simulink model "finalMinhtest3105Part2"  (R2022b)
settings: Solver=VariableStepAuto  StartTime=0.0  StopTime=60  FixedStep=0.001  RelTol=1e-3
undefined symbols (not defined in the file): h, km, m, s, smiData, X, Y, Z
libraries: sm_lib x332, nesl_utility x27, aerolibconvert2 x13, simulink_extras x12, autolibshared x3, simulink x2
(part 1 of 8)
settings Model: Creator=dangm  LastModifiedBy=Lenovo
settings SolverCC: ZeroCrossAlgorithm=Adaptive  AlgebraicLoopSolver=LineSearch
settings DebuggingCC: IgnoredZcDiagnostic=none  UnconnectedInputMsg=warning  UnconnectedOutputMsg=warning  UnconnectedLineMsg=warning  SFMachineParentedDataDiag=warning
settings ModelReferenceCC: EnableRefExpFcnMdlSchedulingChecks=on

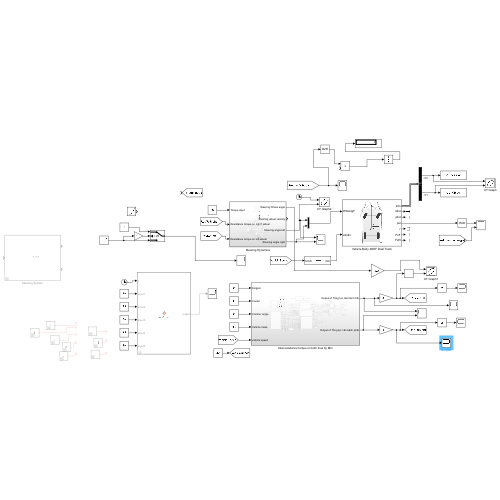
[thumbnail: Simulink's stored preview of the top-level diagram]
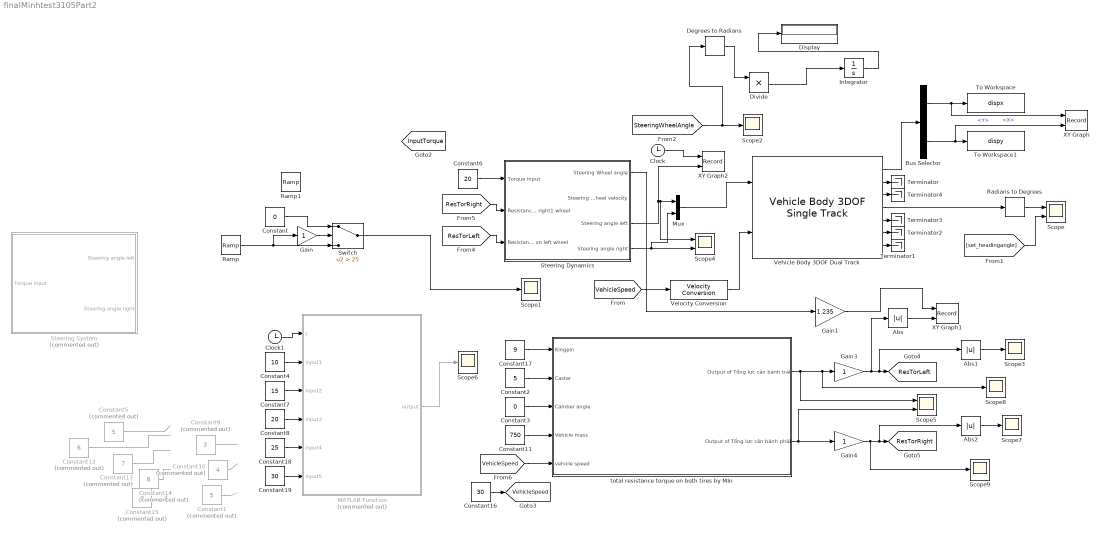
== system finalMinhtest3105Part2 ==
  Abs : Abs  SaturateOnIntegerOverflow=off
  Abs1 : Abs  SaturateOnIntegerOverflow=off
  Abs2 : Abs  SaturateOnIntegerOverflow=off
  Bus Selector : BusSelector  OutputSignals=InertFrm.Cg.Disp.X,InertFrm.Cg.Disp.Y
  Clock : Clock
  Clock1 : Clock
  Constant : Constant  Value=0
  Constant1 : Constant  Commented=on  Value=5
  Constant10 : Constant  Commented=on  Value=4
  Constant11 : Constant  Value=750
  Constant12 : Constant  Commented=on  Value=6
  Constant13 : Constant  Commented=on  Value=7
  Constant14 : Constant  Commented=on  Value=8
  Constant15 : Constant  Commented=on  Value=9
  Constant16 : Constant  Value=30
  Constant17 : Constant  Value=9
  Constant18 : Constant  Value=25
  Constant19 : Constant  Value=30
  Constant2 : Constant  Value=5
  Constant3 : Constant  Value=0
  Constant4 : Constant  Value=10
  Constant5 : Constant  Commented=on  Value=5
  Constant6 : Constant  Value=20
  Constant7 : Constant  Value=15
  Constant8 : Constant  Value=20
  Constant9 : Constant  Commented=on  Value=3
  Degrees to Radians : simulink_extras/Transformations/Degrees to Radians
  Display : Display
  Divide : Product  Inputs=**
  Gain : Gain
  Gain1 : Gain  Gain=1.235
  Gain3 : Gain
  Gain4 : Gain
  Integrator : Integrator
  MATLAB Function : MATLAB Function  Commented=on  TreatAsAtomicUnit=on
  Mux : Mux  Inputs=2
  Radians to Degrees : simulink_extras/Transformations/Radians to Degrees
  Ramp : simulink/Sources/Ramp  slope=1  start=0  InitialOutput=0
  Ramp1 : simulink/Sources/Ramp  slope=0.01  start=0  InitialOutput=0
  Scope : Scope  NumInputPorts=2
  Scope{1..3,6..9} (7 alike) : Scope
  Scope4 : Scope  NumInputPorts=2
  Scope5 : Scope  NumInputPorts=2
  Steering Dynamics : Subsystem
  Steering System : Subsystem  Commented=on
      mask Display: image('D:\MATLAB Projects\MATLAB_EPS_Complete_09_05\CapsoneProject\duy\mask\power-steering-2255498-1882000.png'); % Use "Edit Image" on toolstrip to change.
  Switch : Switch  Criteria=u2 > Threshold  Threshold=25  SaturateOnIntegerOverflow=off  InputSameDT=off
  Terminator{,1..4} (5 alike) : Terminator
  To Workspace : ToWorkspace  VariableName=dispx  SaveFormat=Structure With Time  SampleTime=-1
  To Workspace1 : ToWorkspace  VariableName=dispy  SaveFormat=Structure With Time  SampleTime=-1
  Vehicle Body 3DOF Dual Track : autolibshared/Vehicle Body 3DOF Single Track  trackMode=Dual  inputMode=External longitudinal velocity  frontSteerMode=on  rearSteerMode=off  windMode=off  muMode=off  extFMode=off  extMMode=off  htchFMode=off  htchMMode=off  extXo=off  extpsio=off  extxdoto=off  extro=off  extYo=off  extTamb=off  extydoto=off  aMode=2  NF=2  NR=2  m=1520  a=1.4  b=1.4  h=0.35  dh=1  hh=0.2  X_o=0  xdot_o=0  CalphaMode=off  sigmaMode=on  d=0  hl=0  w=[1.4,1.4]  Cy_f=12e3  Cy_r=11e3  sigma_f=.1  sigma_r=.1  alpha_f_brk=[-.1 .1]  Cy_f_data=[-9e3 9e3]  alpha_r_brk=[-.1 .1]  Cy_r_data=[-9e3 9e3]  Y_o=0  ydot_o=0  Izz=4000  psi_o=0  r_o=0  Af=2  Cd=.3  Cl=.1  Cpm=.1  beta_w=[0:0.01:0.3]  Cs=[0:0.03:0.9]  Cym=[0:0.01:0.3]  Pabs=101325  Tair=273  g=9.81  mu=1  xdot_tol=.01  Fznom=5000  Fxtire_sat=7e4  Fytire_sat=7e4  longOff=0  latOff=0  vertOff=0  wrapAng=off
  Velocity Conversion : aerolibconvert2/Velocity Conversion  IU=km/h  OU=m/s
  XY Graph : Record  FileSettingsInternal="{\"entries\":[{\"content\":{\"excelSettings\":{\"content\":{},\"type\":\"Streamout.ExcelSettings\"}},\"type\":\"Streamout.FileSettingStorage\",\"uuid\":\"8bd62942-ac25-41b1-a812-78b271daa7eb\"}],\"packageUris\":[\"http://schema.mathworks.com/mf0/streamout_blocks/R2020a\"],\"version\":\"1.0\"}"  Layout=[1 1]  SignalsInternal="{\"entries\":[{\"content\":{\"signals\":[{\"content\":{\"blockPath\":[\"FinalTest16_05Long32019b/XY Graph\"],\"channel\":[],\"dimensions\":[1],\"domain\":\"FinalTest16_05Long32019b/XY Graph\",\"lineColor\":\"#a2142f\",\"plots\":[1],\"port\":1,\"sid\":[\"\"],\"signalID\":18325,\"signalName\":\"<X>\"},\"type\":\"RecordBlkView.Signal\",\"uuid\":\"2b0177d6-e985-4d5a-bed9-d4c24acd87c5\"},{\"content\":{\"blockPath\":[\"FinalTest16_05Long32019b/XY Graph\"],\"channel\":[],\"dimensions\":[1],\"domain\":\"FinalTest16_05Long32019b/XY Graph\",\"lineColor\":\"#139fff\",\"plots\":[1],\"port\":2,\"sid\":[\"\"],\"signalID\":18329,\"signalName\":\"<Y>\"},\"type\":\"RecordBlkView.Signal\",\"uuid\":\"3202ecd1-4493-4db3-ae2f-ac69954db6bf\"}]},\"type\":\"RecordBlkView.InputSignals\",\"uuid\":\"6c82ded1-8226-4c26-a1f0-daf373c2f201\"}],\"packageUris\":[\"http://schema.mathworks.com/mf0/streamout_blocks/R2020a\"],\"version\":\"1.0\"}"  VisualizationBindings="{\"xyplotplugin\":{\"info\":[{\"series\":[{\"bindingParametersList\":[{\"parameter\":\"X-Axis\",\"signalID\":18325,\"signalName\":\"<X>\"},{\"parameter\":\"Y-Axis\",\"signalID\":18329,\"signalName\":\"<Y>\"}],\"seriesID\":52564}],\"subplotID\":1}]}}"  CompatibilityTag=XY  st=-1
  XY Graph1 : Record  FileSettingsInternal="{\"entries\":[{\"content\":{\"excelSettings\":{\"content\":{},\"type\":\"Streamout.ExcelSettings\"}},\"type\":\"Streamout.FileSettingStorage\",\"uuid\":\"d249e66b-4ac3-43e9-8db5-f8051359078a\"}],\"packageUris\":[\"http://schema.mathworks.com/mf0/streamout_blocks/R2020a\"],\"version\":\"1.0\"}"  Layout=[1 1]  SignalsInternal="{\"entries\":[{\"content\":{\"signals\":[{\"content\":{\"blockPath\":[\"FinalTest16_05Long32019b/XY Graph1\"],\"channel\":[],\"dimensions\":[1],\"domain\":\"FinalTest16_05Long32019b/XY Graph1\",\"lineColor\":\"#a2142f\",\"plots\":[1],\"port\":1,\"sid\":[\"\"],\"signalID\":18333,\"signalName\":\"Gain1\"},\"type\":\"RecordBlkView.Signal\",\"uuid\":\"ae25a6cb-4a64-4b64-b147-bb834be32e30\"},{\"content\":{\"blockPath\":[\"FinalTest16_05Long32019b/XY Graph1\"],\"channel\":[],\"dimensions\":[1],\"domain\":\"FinalTest16_05Long32019b/XY Graph1\",\"lineColor\":\"#139fff\",\"plots\":[1],\"port\":2,\"sid\":[\"\"],\"signalID\":18337,\"signalName\":\"Abs\"},\"type\":\"RecordBlkView.Signal\",\"uuid\":\"6c87c872-6dc0-4e7a-a83c-45ce04c5dd01\"}]},\"type\":\"RecordBlkView.InputSignals\",\"uuid\":\"a428bf55-466d-414c-9a8e-740befd34512\"}],\"packageUris\":[\"http://schema.mathworks.com/mf0/streamout_blocks/R2020a\"],\"version\":\"1.0\"}"  VisualizationBindings="{\"xyplotplugin\":{\"info\":[{\"series\":[{\"bindingParametersList\":[{\"parameter\":\"X-Axis\",\"signalID\":18333,\"signalName\":\"Gain1\"},{\"parameter\":\"Y-Axis\",\"signalID\":18337,\"signalName\":\"Abs\"}],\"seriesID\":19294}],\"subplotID\":1}]}}"  CompatibilityTag=XY  st=-1
  XY Graph2 : Record  FileSettingsInternal="{\"entries\":[{\"content\":{\"excelSettings\":{\"content\":{},\"type\":\"Streamout.ExcelSettings\"}},\"type\":\"Streamout.FileSettingStorage\",\"uuid\":\"ccaa301e-d718-420b-80cc-2ff8462626e4\"}],\"packageUris\":[\"http://schema.mathworks.com/mf0/streamout_blocks/R2020a\"],\"version\":\"1.0\"}"  Layout=[1 1]  SignalsInternal="{\"entries\":[{\"content\":{\"signals\":[{\"content\":{\"blockPath\":[\"FinalTest16_05Long32019b/XY Graph2\"],\"channel\":[],\"dimensions\":[1],\"domain\":\"FinalTest16_05Long32019b/XY Graph2\",\"lineColor\":\"#a2142f\",\"plots\":[1],\"port\":1,\"sid\":[\"\"],\"signalID\":18341,\"signalName\":\"Clock\"},\"type\":\"RecordBlkView.Signal\",\"uuid\":\"91adbf16-523e-4284-a861-e31794318eab\"},{\"content\":{\"blockPath\":[\"FinalTest16_05Long32019b/XY Graph2\"],\"channel\":[],\"dimensions\":[1],\"domain\":\"FinalTest16_05Long32019b/XY Graph2\",\"lineColor\":\"#139fff\",\"plots\":[1],\"port\":2,\"sid\":[\"\"],\"signalID\":18345,\"signalName\":\"Steering Dynamics:3\"},\"type\":\"RecordBlkView.Signal\",\"uuid\":\"6aaabfaf-cb82-4d42-adb0-24f2f77b8e1f\"}]},\"type\":\"RecordBlkView.InputSignals\",\"uuid\":\"94198bb5-c0f4-4c25-adab-71deb5bd9c4e\"}],\"packageUris\":[\"http://schema.mathworks.com/mf0/streamout_blocks/R2020a\"],\"version\":\"1.0\"}"  VisualizationBindings="{\"xyplotplugin\":{\"info\":[{\"series\":[{\"bindingParametersList\":[{\"parameter\":\"X-Axis\",\"signalID\":18341,\"signalName\":\"Clock\"},{\"parameter\":\"Y-Axis\",\"signalID\":18345,\"signalName\":\"Steering Dynamics:3\"}],\"seriesID\":6618}],\"subplotID\":1}]}}"  CompatibilityTag=XY  st=-1
  total resistance torque on both tires by MIn : Subsystem
  tag scope: InputTorque=global, ResTorLeft=global, ResTorRight=global, VehicleSpeed=global
  wires:
  Mux/1 -> Vehicle Body 3DOF Dual Track/1
  Vehicle Body 3DOF Dual Track/7 -> Terminator1/1
  Vehicle Body 3DOF Dual Track/6 -> Terminator2/1
  Vehicle Body 3DOF Dual Track/5 -> Terminator3/1
  Vehicle Body 3DOF Dual Track/1 -> Bus Selector/1
  Bus Selector/1 -> XY Graph/1, To Workspace/1  "<X>"
  Bus Selector/2 -> XY Graph/2, To Workspace1/1  "<Y>"
  Velocity Conversion/1 -> Vehicle Body 3DOF Dual Track/2
  [VehicleSpeed] -> Velocity Conversion/1
  Vehicle Body 3DOF Dual Track/2 -> Terminator/1
  Vehicle Body 3DOF Dual Track/3 -> Terminator4/1
  Vehicle Body 3DOF Dual Track/4 -> Radians to Degrees/1
  Radians to Degrees/1 -> Scope/1
  [set_headingangle] -> Scope/2
  [SteeringWheelAngle] -> Scope2/1, Degrees to Radians/1
  Gain4/1 -> Scope9/1, Abs2/1, [ResTorRight]
  total resistance torque on both tires by MIn/1(Output of Tổng lực cản bánh trái) -> Scope5/1, Scope8/1, Gain3/1
  total resistance torque on both tires by MIn/2(Output of Tổng lực cản bánh phải) -> Gain4/1, Scope5/2
  Degrees to Radians/1 -> Divide/1
  Divide/1 -> Integrator/1
  Integrator/1 -> Display/1
  Constant/1 -> Switch/1
  Ramp/1 -> Gain/1, Switch/3
  Steering Dynamics/3(Steering angle left) -> XY Graph2/2, Scope4/1, Mux/1
  Steering Dynamics/4(Steering angle right) -> Mux/2, Scope4/2
  [ResTorRight] -> Steering Dynamics/2(Resistance torque on right1 wheel)
  [ResTorLeft] -> Steering Dynamics/3(Resistance torque on left wheel)
  Steering Dynamics/1(Steering Wheel angle) -> Gain1/1
  Gain/1 -> Switch/2
  Abs/1 -> XY Graph1/2
  Gain1/1 -> XY Graph1/1
  Clock/1 -> XY Graph2/1
  Clock1/1 -> MATLAB Function/1(t)
  Constant4/1 -> MATLAB Function/2(input1)
  Constant7/1 -> MATLAB Function/3(input2)
  Constant8/1 -> MATLAB Function/4(input3)
  Constant10/1 -> ?
  Switch/1 -> Scope1/1
  Gain3/1 -> Abs/1, Abs1/1, [ResTorLeft]
  Constant5/1 -> ?
  Constant12/1 -> ?
  Constant13/1 -> ?
  Constant14/1 -> ?
  Constant15/1 -> ?
  Constant9/1 -> ?
  Constant17/1 -> total resistance torque on both tires by MIn/1(Kingpin)
  Constant11/1 -> total resistance torque on both tires by MIn/4(Vehicle mass)
  Constant1/1 -> ?
  MATLAB Function/1(output) -> Scope6/1
  Abs1/1 -> Scope3/1
  Abs2/1 -> Scope7/1
  Constant2/1 -> total resistance torque on both tires by MIn/2(Caster)
  Constant3/1 -> total resistance torque on both tires by MIn/3(Camber angle)
  Constant18/1 -> MATLAB Function/5(input4)
  Constant19/1 -> MATLAB Function/6(input5)
  Constant16/1 -> [VehicleSpeed]
  [VehicleSpeed] -> total resistance torque on both tires by MIn/5("vehicle speed ")
  Constant6/1 -> Steering Dynamics/1(Torque input)

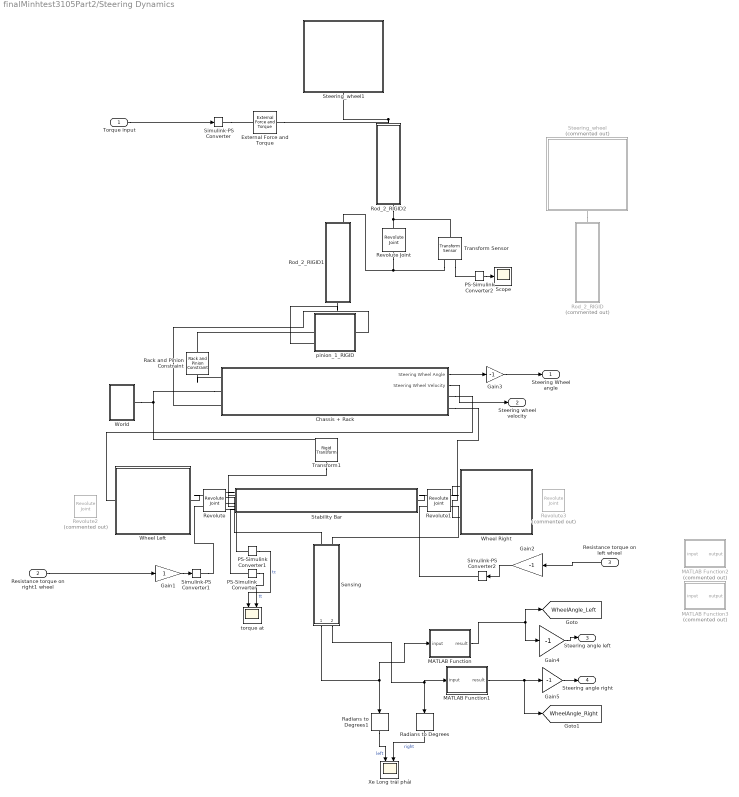
== system finalMinhtest3105Part2/Steering Dynamics ==
  Torque input : Inport
  Resistance torque on right1 wheel : Inport  Port=2
  Resistance torque on left wheel : Inport  Port=3
  Chassis + Rack : Subsystem
      mask Display: image('$imagefile'); % Use "Edit Image" on toolstrip to change.
  External Force and Torque : sm_lib/Forces and Torques/External Force and Torque  ForceResolutionFrame=AttachedFrame  EnableForceX=off  EnableForceY=off  EnableForceZ=off  EnableForce=off  TorqueResolutionFrame=AttachedFrame  EnableTorqueX=off  EnableTorqueY=off  EnableTorqueZ=on  EnableTorque=off
  Gain1 : Gain
  Gain{2..5} (4 alike) : Gain  Gain=-1
  MATLAB Function : MATLAB Function  TreatAsAtomicUnit=on
  MATLAB Function1 : MATLAB Function  TreatAsAtomicUnit=on
  MATLAB Function2 : MATLAB Function  Commented=on  TreatAsAtomicUnit=on
  MATLAB Function3 : MATLAB Function  Commented=on  TreatAsAtomicUnit=on
  PS-Simulink Converter : nesl_utility/PS-Simulink Converter  PhysicalDomain=network_engine_domain  SubClassName=ps_output  LeftPortType=input  RightPortType=output  PseudoPeriodic=off  Frequencies=[]  VectorFormat=1-D array  Unit=inherit  AffineConversion=off
  PS-Simulink Converter1 : nesl_utility/PS-Simulink Converter  PhysicalDomain=network_engine_domain  SubClassName=ps_output  LeftPortType=input  RightPortType=output  PseudoPeriodic=off  Frequencies=[]  VectorFormat=1-D array  Unit=inherit  AffineConversion=off
  PS-Simulink Converter2 : nesl_utility/PS-Simulink Converter  PhysicalDomain=network_engine_domain  SubClassName=ps_output  LeftPortType=input  RightPortType=output  PseudoPeriodic=off  Frequencies=[]  VectorFormat=inherit  Unit=inherit  AffineConversion=off
  Rack and Pinion Constraint : sm_lib/Gears and Couplings/Gears/Rack and Pinion Constraint  PinionRadius=30  PinionRadiusUnits=mm
  Radians to Degrees : simulink_extras/Transformations/Radians to Degrees
  Radians to Degrees1 : simulink_extras/Transformations/Radians to Degrees
  Revolute : sm_lib/Joints/Revolute Joint  JointMode=Normal  SenseConstraintForce=off  SenseConstraintForceX=off  SenseConstraintForceY=off  SenseConstraintForceZ=off  SenseConstraintTorque=on  SenseConstraintTorqueX=off  SenseConstraintTorqueY=off  SenseConstraintTorqueZ=off  SenseTotalForce=off  SenseTotalForceX=off  SenseTotalForceY=off  SenseTotalForceZ=off  SenseTotalTorque=on  SenseTotalTorqueX=off  SenseTotalTorqueY=off  SenseTotalTorqueZ=off  CompositeWrenchDir=BaseOnFollower  CompositeWrenchFrame=FollowerFrame  EquilibriumPosition=0  EquilibriumPositionUnits=deg  SpringStiffness=0.0524-0.0524  SpringStiffnessUnits=N*m/deg  DampingCoefficient=1.5-1.5+0.1  DampingCoefficientUnits=N*m/(deg/s)  TorqueActuationMode=InputTorque  MotionActuationMode=ComputedMotion  SensePosition=on  SenseVelocity=off  SenseAcceleration=off  SenseTorqueForce=off  SenseLowerLimitTorqueForce=off  SenseUpperLimitTorqueForce=off  LowerLimitSpecify=on  LowerLimitBound=-89.68-28.95  LowerLimitBoundUnits=deg  LowerLimitStiffness=1e4  LowerLimitStiffnessUnits=N*m/deg  LowerLimitDamping=100  LowerLimitDampingUnits=N*m/(deg/s)  LowerLimitTransitionRegionWidth=0.1  LowerLimitTransitionRegionWidthUnits=deg  UpperLimitSpecify=on  UpperLimitBound=-89.68+18.80  UpperLimitBoundUnits=deg  UpperLimitStiffness=1e4  UpperLimitStiffnessUnits=N*m/deg  UpperLimitDamping=100  UpperLimitDampingUnits=N*m/(deg/s)  UpperLimitTransitionRegionWidth=0.1  UpperLimitTransitionRegionWidthUnits=deg  PositionTargetSpecify=on  PositionTargetPriority=High  PositionTargetValue=-89.678329494  PositionTargetValueUnits=deg  VelocityTargetSpecify=on  VelocityTargetPriority=High  VelocityTargetValue=0  VelocityTargetValueUnits=deg/s
  Revolute Joint : sm_lib/Joints/Revolute Joint  JointMode=Normal  SenseConstraintForce=off  SenseConstraintForceX=off  SenseConstraintForceY=off  SenseConstraintForceZ=off  SenseConstraintTorque=off  SenseConstraintTorqueX=off  SenseConstraintTorqueY=off  SenseConstraintTorqueZ=off  SenseTotalForce=off  SenseTotalForceX=off  SenseTotalForceY=off  SenseTotalForceZ=off  SenseTotalTorque=off  SenseTotalTorqueX=off  SenseTotalTorqueY=off  SenseTotalTorqueZ=off  CompositeWrenchDir=FollowerOnBase  CompositeWrenchFrame=BaseFrame  EquilibriumPosition=0  EquilibriumPositionUnits=deg  SpringStiffness=10  SpringStiffnessUnits=N*m/deg  DampingCoefficient=1  DampingCoefficientUnits=N*m/(deg/s)  TorqueActuationMode=NoTorque  MotionActuationMode=ComputedMotion  SensePosition=off  SenseVelocity=off  SenseAcceleration=off  SenseTorqueForce=off  SenseLowerLimitTorqueForce=off  SenseUpperLimitTorqueForce=off  LowerLimitSpecify=off  LowerLimitBound=-90  LowerLimitBoundUnits=deg  LowerLimitStiffness=1e4  LowerLimitStiffnessUnits=N*m/deg  LowerLimitDamping=10  LowerLimitDampingUnits=N*m/(deg/s)  LowerLimitTransitionRegionWidth=0.1  LowerLimitTransitionRegionWidthUnits=deg  UpperLimitSpecify=off  UpperLimitBound=90  UpperLimitBoundUnits=deg  UpperLimitStiffness=1e4  UpperLimitStiffnessUnits=N*m/deg  UpperLimitDamping=10  UpperLimitDampingUnits=N*m/(deg/s)  UpperLimitTransitionRegionWidth=0.1  UpperLimitTransitionRegionWidthUnits=deg  PositionTargetSpecify=off  PositionTargetPriority=High  PositionTargetValue=0  PositionTargetValueUnits=deg  VelocityTargetSpecify=off  VelocityTargetPriority=High  VelocityTargetValue=0  VelocityTargetValueUnits=deg/s
  Revolute1 : sm_lib/Joints/Revolute Joint  JointMode=Normal  SenseConstraintForce=off  SenseConstraintForceX=off  SenseConstraintForceY=off  SenseConstraintForceZ=off  SenseConstraintTorque=off  SenseConstraintTorqueX=off  SenseConstraintTorqueY=off  SenseConstraintTorqueZ=off  SenseTotalForce=off  SenseTotalForceX=off  SenseTotalForceY=off  SenseTotalForceZ=off  SenseTotalTorque=off  SenseTotalTorqueX=off  SenseTotalTorqueY=off  SenseTotalTorqueZ=off  CompositeWrenchDir=FollowerOnBase  CompositeWrenchFrame=FollowerFrame  EquilibriumPosition=0  EquilibriumPositionUnits=deg  SpringStiffness=0  SpringStiffnessUnits=N*m/deg  DampingCoefficient=0.1  DampingCoefficientUnits=N*m/(deg/s)  TorqueActuationMode=InputTorque  MotionActuationMode=ComputedMotion  SensePosition=on  SenseVelocity=off  SenseAcceleration=off  SenseTorqueForce=off  SenseLowerLimitTorqueForce=off  SenseUpperLimitTorqueForce=off  LowerLimitSpecify=on  LowerLimitBound=-89.68-28.95  LowerLimitBoundUnits=deg  LowerLimitStiffness=1e4  LowerLimitStiffnessUnits=N*m/deg  LowerLimitDamping=100  LowerLimitDampingUnits=N*m/(deg/s)  LowerLimitTransitionRegionWidth=0.1  LowerLimitTransitionRegionWidthUnits=deg  UpperLimitSpecify=on  UpperLimitBound=-89.68+18.80  UpperLimitBoundUnits=deg  UpperLimitStiffness=1e4  UpperLimitStiffnessUnits=N*m/deg  UpperLimitDamping=100  UpperLimitDampingUnits=N*m/(deg/s)  UpperLimitTransitionRegionWidth=0.1  UpperLimitTransitionRegionWidthUnits=deg  PositionTargetSpecify=on  PositionTargetPriority=Low  PositionTargetValue=smiData.RevoluteJoint(2).Rz.Pos-2.7  PositionTargetValueUnits=deg  VelocityTargetSpecify=on  VelocityTargetPriority=High  VelocityTargetValue=0  VelocityTargetValueUnits=deg/s
  Revolute2 : sm_lib/Joints/Revolute Joint  Commented=on  JointMode=Normal  SenseConstraintForce=off  SenseConstraintForceX=off  SenseConstraintForceY=off  SenseConstraintForceZ=off  SenseConstraintTorque=off  SenseConstraintTorqueX=off  SenseConstraintTorqueY=off  SenseConstraintTorqueZ=off  SenseTotalForce=off  SenseTotalForceX=off  SenseTotalForceY=off  SenseTotalForceZ=off  SenseTotalTorque=off  SenseTotalTorqueX=off  SenseTotalTorqueY=off  SenseTotalTorqueZ=off  CompositeWrenchDir=BaseOnFollower  CompositeWrenchFrame=FollowerFrame  EquilibriumPosition=0  EquilibriumPositionUnits=deg  SpringStiffness=0.0524-0.0524+0.1  SpringStiffnessUnits=N*m/deg  DampingCoefficient=1.5-1.5+0.1  DampingCoefficientUnits=N*m/(deg/s)  TorqueActuationMode=InputTorque  MotionActuationMode=ComputedMotion  SensePosition=on  SenseVelocity=off  SenseAcceleration=off  SenseTorqueForce=off  SenseLowerLimitTorqueForce=off  SenseUpperLimitTorqueForce=off  LowerLimitSpecify=on  LowerLimitBound=-2+0.089+0.071  LowerLimitBoundUnits=rad  LowerLimitStiffness=1e4  LowerLimitStiffnessUnits=N*m/deg  LowerLimitDamping=100  LowerLimitDampingUnits=N*m/(deg/s)  LowerLimitTransitionRegionWidth=0.1  LowerLimitTransitionRegionWidthUnits=deg  UpperLimitSpecify=on  UpperLimitBound=-1-0.195-0.106  UpperLimitBoundUnits=rad  UpperLimitStiffness=1e4  UpperLimitStiffnessUnits=N*m/deg  UpperLimitDamping=100  UpperLimitDampingUnits=N*m/(deg/s)  UpperLimitTransitionRegionWidth=0.1  UpperLimitTransitionRegionWidthUnits=deg  PositionTargetSpecify=on  PositionTargetPriority=High  PositionTargetValue=-89.678329494  PositionTargetValueUnits=deg  VelocityTargetSpecify=on  VelocityTargetPriority=High  VelocityTargetValue=0  VelocityTargetValueUnits=deg/s
  Revolute3 : sm_lib/Joints/Revolute Joint  Commented=on  JointMode=Normal  SenseConstraintForce=off  SenseConstraintForceX=off  SenseConstraintForceY=off  SenseConstraintForceZ=off  SenseConstraintTorque=off  SenseConstraintTorqueX=off  SenseConstraintTorqueY=off  SenseConstraintTorqueZ=off  SenseTotalForce=off  SenseTotalForceX=off  SenseTotalForceY=off  SenseTotalForceZ=off  SenseTotalTorque=off  SenseTotalTorqueX=off  SenseTotalTorqueY=off  SenseTotalTorqueZ=off  CompositeWrenchDir=FollowerOnBase  CompositeWrenchFrame=FollowerFrame  EquilibriumPosition=0  EquilibriumPositionUnits=deg  SpringStiffness=0.1  SpringStiffnessUnits=N*m/deg  DampingCoefficient=0.1  DampingCoefficientUnits=N*m/(deg/s)  TorqueActuationMode=InputTorque  MotionActuationMode=ComputedMotion  SensePosition=on  SenseVelocity=off  SenseAcceleration=off  SenseTorqueForce=off  SenseLowerLimitTorqueForce=off  SenseUpperLimitTorqueForce=off  LowerLimitSpecify=off  LowerLimitBound=-2  LowerLimitBoundUnits=rad  LowerLimitStiffness=1e4  LowerLimitStiffnessUnits=N*m/deg  LowerLimitDamping=100  LowerLimitDampingUnits=N*m/(deg/s)  LowerLimitTransitionRegionWidth=0.1  LowerLimitTransitionRegionWidthUnits=deg  UpperLimitSpecify=off  UpperLimitBound=-1  UpperLimitBoundUnits=rad  UpperLimitStiffness=1e4  UpperLimitStiffnessUnits=N*m/deg  UpperLimitDamping=100  UpperLimitDampingUnits=N*m/(deg/s)  UpperLimitTransitionRegionWidth=0.1  UpperLimitTransitionRegionWidthUnits=deg  PositionTargetSpecify=on  PositionTargetPriority=Low  PositionTargetValue=smiData.RevoluteJoint(2).Rz.Pos-2.7  PositionTargetValueUnits=deg  VelocityTargetSpecify=on  VelocityTargetPriority=High  VelocityTargetValue=0  VelocityTargetValueUnits=deg/s
  Rod_2_RIGID : Subsystem  Commented=on
      mask Display: image('rod.png'); % Use "Edit Image" on toolstrip to change.
  Rod_2_RIGID1 : Subsystem
  Rod_2_RIGID2 : Subsystem
  Scope : Scope
  "Sensing " : Subsystem
  Simulink-PS Converter : nesl_utility/Simulink-PS Converter  PhysicalDomain=network_engine_domain  SubClassName=ps_input  LeftPortType=input  RightPortType=output  PseudoPeriodic=off  Frequencies=[]  NoiseDistribution=none  NoiseParameters=[]  Unit=N*m  AffineConversion=off  FilteringAndDerivatives=provide  SimscapeFilterOrder=1  InputFilterTimeConstant=0.001  UdotUserProvided=0
  Simulink-PS Converter1 : nesl_utility/Simulink-PS Converter  PhysicalDomain=network_engine_domain  SubClassName=ps_input  LeftPortType=input  RightPortType=output  PseudoPeriodic=off  Frequencies=[]  NoiseDistribution=none  NoiseParameters=[]  Unit=N*m  AffineConversion=off  FilteringAndDerivatives=provide  SimscapeFilterOrder=1  InputFilterTimeConstant=0.001  UdotUserProvided=0
  Simulink-PS Converter2 : nesl_utility/Simulink-PS Converter  PhysicalDomain=network_engine_domain  SubClassName=ps_input  LeftPortType=input  RightPortType=output  PseudoPeriodic=off  Frequencies=[]  NoiseDistribution=none  NoiseParameters=[]  Unit=N*m  AffineConversion=off  FilteringAndDerivatives=provide  SimscapeFilterOrder=2  InputFilterTimeConstant=0.001  UdotUserProvided=0
  Stability Bar : Subsystem
      mask Display: image('$imagefile'); % Use "Edit Image" on toolstrip to change.
  Steering_wheel : Subsystem  Commented=on
      mask Display: image('$imagefile'); % Use "Edit Image" on toolstrip to change.
  Steering_wheel1 : Subsystem
      mask Display: image('$imagefile'); % Use "Edit Image" on toolstrip to change.
  Transform Sensor : sm_lib/Frames and Transforms/Transform Sensor  MeasurementFrame=Base  SenseAngle=on  SenseAxis=off  SenseQ=off  SenseR=off  SenseRotationSequence=off  RotationSequence=XYX  SenseOmegaX=off  SenseOmegaY=off  SenseOmegaZ=off  SenseQDot=off  SenseRDot=off  SenseAlphaX=off  SenseAlphaY=off  SenseAlphaZ=off  SenseQDDot=off  SenseRDDot=off  SenseX=off  SenseY=off  SenseZ=off  SenseRad=off  SenseAzim=off  SenseDist=off  SenseInc=off  SenseXDot=off  SenseYDot=off  SenseZDot=off  SenseRadDot=off  SenseAzimDot=off  SenseDistDot=off  SenseIncDot=off  SenseXDDot=off  SenseYDDot=off  SenseZDDot=off  SenseRadDDot=off  SenseAzimDDot=off  SenseDistDDot=off  SenseIncDDot=off
  Transform1 : sm_lib/Frames and Transforms/Rigid Transform  TranslationMethod=Cartesian  TranslationStandardOffset=0  TranslationLengthUnit=mm  TranslationStandardAxis=+Z  TranslationCartesianOffset=smiData.RigidTransform(48).translation  TranslationROffset=0  TranslationROffsetUnits=m  TranslationZOffset=0  TranslationZOffsetUnits=m  TranslationThetaOffset=0  TranslationThetaOffsetUnits=deg  RotationMethod=ArbitraryAxis  RotationAngleUnits=rad  RotationStandardAxis=+Z  RotationAngle=smiData.RigidTransform(48).angle  RotationArbitraryAxis=smiData.RigidTransform(48).axis  FollAlignAxisA=+X  BaseAlignAxisA=+Y  FollAlignAxisB=+Y  BaseAlignAxisB=+Z  RotationSequenceAxes=FollowerAxes  RotationSequence=XYX  RotationSequenceAngles=[0 0 0]  RotationSequenceAnglesUnits=deg  RotationMatrix=[1 0 0; 0 1 0; 0 0 1]  Quaternion=[1 0 0 0]
  Wheel Left : Subsystem
      mask Display: image('$imagefile'); % Use "Edit Image" on toolstrip to change.
  Wheel Right : Subsystem
      mask Display: image('$imagefile'); % Use "Edit Image" on toolstrip to change.
  World : Subsystem
  Xe Long trái phải : Scope  NumInputPorts=2
  pinion_1_RIGID : Subsystem
      mask Display: image('pinion.png'); % Use "Edit Image" on toolstrip to change.
  "torque at " : Scope  NumInputPorts=2
  Steering Wheel angle : Outport
  Steering wheel velocity : Outport  Port=2
  Steering angle left : Outport  Port=3
  Steering angle right : Outport  Port=4
  tag scope: WheelAngle_Left=global, WheelAngle_Right=global
  wires:
  "Sensing "/2(Steering angle right (rad)) -> MATLAB Function1/1(input), Radians to Degrees/1
  Radians to Degrees/1 -> Xe Long trái phải/2  "right"
  Radians to Degrees1/1 -> Xe Long trái phải/1  "left"
  Chassis + Rack/2(Steering Wheel Velocity) -> Steering wheel velocity/1
  Chassis + Rack/1(Steering Wheel Angle) -> Gain3/1
  Resistance torque on right1 wheel/1 -> Gain1/1
  Resistance torque on left wheel/1 -> Gain2/1
  Gain1/1 -> Simulink-PS Converter1/1
  Gain2/1 -> Simulink-PS Converter2/1
  MATLAB Function/1(result) -> Gain4/1, [WheelAngle_Left]
  MATLAB Function1/1(result) -> [WheelAngle_Right], Gain5/1
  "Sensing "/1(Steering angle left (rad)) -> Radians to Degrees1/1, MATLAB Function/1(input)
  PS-Simulink Converter1/1 -> "torque at "/1  "tc"
  PS-Simulink Converter/1 -> "torque at "/2  "tt"
  Torque input/1 -> Simulink-PS Converter/1
  Gain3/1 -> Steering Wheel angle/1
  PS-Simulink Converter2/1 -> Scope/1
  Gain4/1 -> Steering angle left/1
  Gain5/1 -> Steering angle right/1
  connections:
  Revolute/RConn2 -- "Sensing "/LConn1
  Simulink-PS Converter/RConn1 -- External Force and Torque/LConn1
  Chassis + Rack/LConn2 -- World/LConn1 -- Transform1/LConn1
  Rack and Pinion Constraint/RConn1 -- Chassis + Rack/LConn1
  Revolute1/RConn2 -- "Sensing "/LConn2
  Rack and Pinion Constraint/LConn1 -- pinion_1_RIGID/LConn2
  Transform1/RConn1 -- Stability Bar/LConn2
  Chassis + Rack/LConn3 -- pinion_1_RIGID/RConn1
  Chassis + Rack/RConn1 -- Wheel Left/LConn1
  Revolute1/RConn1 -- Wheel Right/LConn1
  Chassis + Rack/RConn2 -- Wheel Right/LConn2
  Revolute1/LConn1 -- Stability Bar/RConn1
  Revolute/RConn1 -- Stability Bar/LConn1
  Revolute/LConn1 -- Wheel Left/RConn1
  Rod_2_RIGID1/RConn1 -- pinion_1_RIGID/LConn3
  Steering_wheel/LConn1 -- Rod_2_RIGID/LConn1
  Simulink-PS Converter1/RConn1 -- Revolute/LConn2
  Revolute1/LConn2 -- Simulink-PS Converter2/RConn1
  Revolute/RConn3 -- PS-Simulink Converter1/LConn1
  Revolute/RConn4 -- PS-Simulink Converter/LConn1
  Steering_wheel1/LConn1 -- External Force and Torque/RConn1 -- Rod_2_RIGID2/LConn1
  Revolute Joint/RConn1 -- Transform Sensor/RConn1 -- Rod_2_RIGID1/LConn2
  Rod_2_RIGID2/RConn2 -- Transform Sensor/LConn1 -- Revolute Joint/LConn1
  Transform Sensor/RConn2 -- PS-Simulink Converter2/LConn1

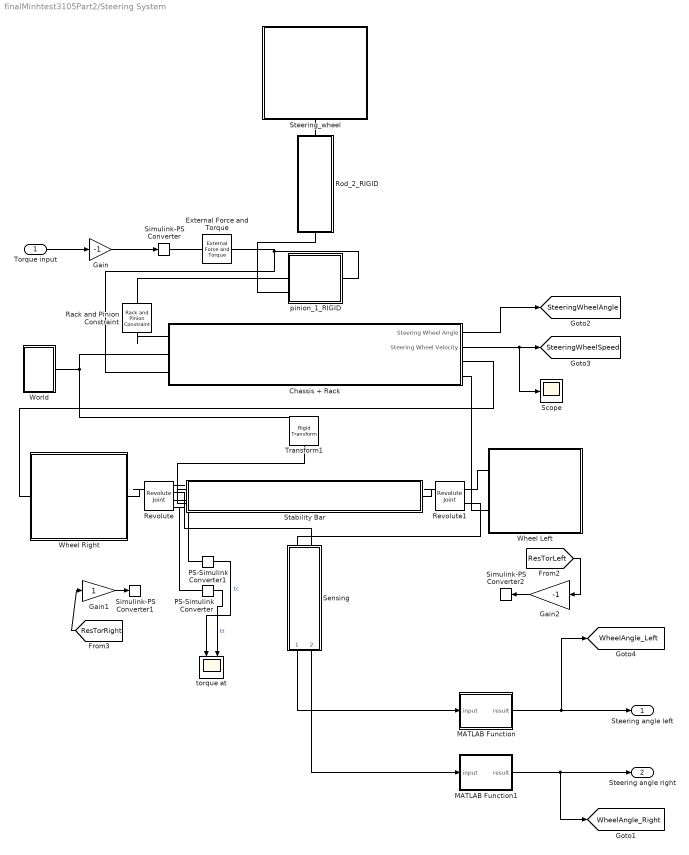
== system finalMinhtest3105Part2/Steering System ==
  Torque input : Inport
  Chassis + Rack : Subsystem
      mask Display: image('$imagefile'); % Use "Edit Image" on toolstrip to change.
  External Force and Torque : sm_lib/Forces and Torques/External Force and Torque  ForceResolutionFrame=AttachedFrame  EnableForceX=off  EnableForceY=off  EnableForceZ=off  EnableForce=off  TorqueResolutionFrame=AttachedFrame  EnableTorqueX=off  EnableTorqueY=off  EnableTorqueZ=on  EnableTorque=off
  Gain : Gain  Gain=-1
  Gain1 : Gain
  Gain2 : Gain  Gain=-1
  MATLAB Function : MATLAB Function  TreatAsAtomicUnit=on
  MATLAB Function1 : MATLAB Function  TreatAsAtomicUnit=on
  PS-Simulink Converter : nesl_utility/PS-Simulink Converter  PhysicalDomain=network_engine_domain  SubClassName=ps_output  LeftPortType=input  RightPortType=output  PseudoPeriodic=off  Frequencies=[]  VectorFormat=1-D array  Unit=inherit  AffineConversion=off
  PS-Simulink Converter1 : nesl_utility/PS-Simulink Converter  PhysicalDomain=network_engine_domain  SubClassName=ps_output  LeftPortType=input  RightPortType=output  PseudoPeriodic=off  Frequencies=[]  VectorFormat=1-D array  Unit=inherit  AffineConversion=off
  Rack and Pinion Constraint : sm_lib/Gears and Couplings/Gears/Rack and Pinion Constraint  PinionRadius=30  PinionRadiusUnits=mm
  Revolute : sm_lib/Joints/Revolute Joint  JointMode=Normal  SenseConstraintForce=off  SenseConstraintForceX=off  SenseConstraintForceY=off  SenseConstraintForceZ=off  SenseConstraintTorque=on  SenseConstraintTorqueX=off  SenseConstraintTorqueY=off  SenseConstraintTorqueZ=off  SenseTotalForce=off  SenseTotalForceX=off  SenseTotalForceY=off  SenseTotalForceZ=off  SenseTotalTorque=on  SenseTotalTorqueX=off  SenseTotalTorqueY=off  SenseTotalTorqueZ=off  CompositeWrenchDir=BaseOnFollower  CompositeWrenchFrame=FollowerFrame  EquilibriumPosition=0  EquilibriumPositionUnits=deg  SpringStiffness=0.0524-0.0524+0.1  SpringStiffnessUnits=N*m/deg  DampingCoefficient=1.5-1.5+0.1  DampingCoefficientUnits=N*m/(deg/s)  TorqueActuationMode=InputTorque  MotionActuationMode=ComputedMotion  SensePosition=on  SenseVelocity=off  SenseAcceleration=off  SenseTorqueForce=off  SenseLowerLimitTorqueForce=off  SenseUpperLimitTorqueForce=off  LowerLimitSpecify=on  LowerLimitBound=-89.68-28.95  LowerLimitBoundUnits=deg  LowerLimitStiffness=1e4  LowerLimitStiffnessUnits=N*m/deg  LowerLimitDamping=100  LowerLimitDampingUnits=N*m/(deg/s)  LowerLimitTransitionRegionWidth=0.1  LowerLimitTransitionRegionWidthUnits=deg  UpperLimitSpecify=on  UpperLimitBound=-89.68+18.80  UpperLimitBoundUnits=deg  UpperLimitStiffness=1e4  UpperLimitStiffnessUnits=N*m/deg  UpperLimitDamping=100  UpperLimitDampingUnits=N*m/(deg/s)  UpperLimitTransitionRegionWidth=0.1  UpperLimitTransitionRegionWidthUnits=deg  PositionTargetSpecify=on  PositionTargetPriority=High  PositionTargetValue=-89.678329494  PositionTargetValueUnits=deg  VelocityTargetSpecify=on  VelocityTargetPriority=High  VelocityTargetValue=0  VelocityTargetValueUnits=deg/s
  Revolute1 : sm_lib/Joints/Revolute Joint  JointMode=Normal  SenseConstraintForce=off  SenseConstraintForceX=off  SenseConstraintForceY=off  SenseConstraintForceZ=off  SenseConstraintTorque=off  SenseConstraintTorqueX=off  SenseConstraintTorqueY=off  SenseConstraintTorqueZ=off  SenseTotalForce=off  SenseTotalForceX=off  SenseTotalForceY=off  SenseTotalForceZ=off  SenseTotalTorque=off  SenseTotalTorqueX=off  SenseTotalTorqueY=off  SenseTotalTorqueZ=off  CompositeWrenchDir=FollowerOnBase  CompositeWrenchFrame=FollowerFrame  EquilibriumPosition=0  EquilibriumPositionUnits=deg  SpringStiffness=0.1  SpringStiffnessUnits=N*m/deg  DampingCoefficient=0.1  DampingCoefficientUnits=N*m/(deg/s)  TorqueActuationMode=InputTorque  MotionActuationMode=ComputedMotion  SensePosition=on  SenseVelocity=off  SenseAcceleration=off  SenseTorqueForce=off  SenseLowerLimitTorqueForce=off  SenseUpperLimitTorqueForce=off  LowerLimitSpecify=on  LowerLimitBound=-89.68-28.95  LowerLimitBoundUnits=deg  LowerLimitStiffness=1e4  LowerLimitStiffnessUnits=N*m/deg  LowerLimitDamping=100  LowerLimitDampingUnits=N*m/(deg/s)  LowerLimitTransitionRegionWidth=0.1  LowerLimitTransitionRegionWidthUnits=deg  UpperLimitSpecify=on  UpperLimitBound=-89.68+18.80  UpperLimitBoundUnits=deg  UpperLimitStiffness=1e4  UpperLimitStiffnessUnits=N*m/deg  UpperLimitDamping=100  UpperLimitDampingUnits=N*m/(deg/s)  UpperLimitTransitionRegionWidth=0.1  UpperLimitTransitionRegionWidthUnits=deg  PositionTargetSpecify=on  PositionTargetPriority=Low  PositionTargetValue=smiData.RevoluteJoint(2).Rz.Pos-2.7  PositionTargetValueUnits=deg  VelocityTargetSpecify=on  VelocityTargetPriority=High  VelocityTargetValue=0  VelocityTargetValueUnits=deg/s
  Rod_2_RIGID : Subsystem
      mask Display: image('rod.png'); % Use "Edit Image" on toolstrip to change.
  Scope : Scope
  "Sensing " : Subsystem
  Simulink-PS Converter : nesl_utility/Simulink-PS Converter  PhysicalDomain=network_engine_domain  SubClassName=ps_input  LeftPortType=input  RightPortType=output  PseudoPeriodic=off  Frequencies=[]  NoiseDistribution=none  NoiseParameters=[]  Unit=N*m  AffineConversion=off  FilteringAndDerivatives=provide  SimscapeFilterOrder=1  InputFilterTimeConstant=0.001  UdotUserProvided=0
  Simulink-PS Converter1 : nesl_utility/Simulink-PS Converter  PhysicalDomain=network_engine_domain  SubClassName=ps_input  LeftPortType=input  RightPortType=output  PseudoPeriodic=off  Frequencies=[]  NoiseDistribution=none  NoiseParameters=[]  Unit=N*m  AffineConversion=off  FilteringAndDerivatives=provide  SimscapeFilterOrder=1  InputFilterTimeConstant=0.001  UdotUserProvided=0
  Simulink-PS Converter2 : nesl_utility/Simulink-PS Converter  PhysicalDomain=network_engine_domain  SubClassName=ps_input  LeftPortType=input  RightPortType=output  PseudoPeriodic=off  Frequencies=[]  NoiseDistribution=none  NoiseParameters=[]  Unit=N*m  AffineConversion=off  FilteringAndDerivatives=provide  SimscapeFilterOrder=2  InputFilterTimeConstant=0.001  UdotUserProvided=0
  Stability Bar : Subsystem
      mask Display: image('$imagefile'); % Use "Edit Image" on toolstrip to change.
  Steering_wheel : Subsystem
      mask Display: image('$imagefile'); % Use "Edit Image" on toolstrip to change.
  Transform1 : sm_lib/Frames and Transforms/Rigid Transform  TranslationMethod=Cartesian  TranslationStandardOffset=0  TranslationLengthUnit=mm  TranslationStandardAxis=+Z  TranslationCartesianOffset=smiData.RigidTransform(48).translation  TranslationROffset=0  TranslationROffsetUnits=m  TranslationZOffset=0  TranslationZOffsetUnits=m  TranslationThetaOffset=0  TranslationThetaOffsetUnits=deg  RotationMethod=ArbitraryAxis  RotationAngleUnits=rad  RotationStandardAxis=+Z  RotationAngle=smiData.RigidTransform(48).angle  RotationArbitraryAxis=smiData.RigidTransform(48).axis  FollAlignAxisA=+X  BaseAlignAxisA=+Y  FollAlignAxisB=+Y  BaseAlignAxisB=+Z  RotationSequenceAxes=FollowerAxes  RotationSequence=XYX  RotationSequenceAngles=[0 0 0]  RotationSequenceAnglesUnits=deg  RotationMatrix=[1 0 0; 0 1 0; 0 0 1]  Quaternion=[1 0 0 0]
  Wheel Left : Subsystem
      mask Display: image('$imagefile'); % Use "Edit Image" on toolstrip to change.
  Wheel Right : Subsystem
      mask Display: image('$imagefile'); % Use "Edit Image" on toolstrip to change.
  World : Subsystem
  pinion_1_RIGID : Subsystem
  "torque at " : Scope  NumInputPorts=2
  Steering angle left : Outport
  Steering angle right : Outport  Port=2
  tag scope: SteeringWheelAngle=global, SteeringWheelSpeed=global, WheelAngle_Left=global, WheelAngle_Right=global
  wires:
  "Sensing "/2(Steering angle right (rad)) -> MATLAB Function1/1(input)
  Chassis + Rack/2(Steering Wheel Velocity) -> Scope/1, [SteeringWheelSpeed]
  Chassis + Rack/1(Steering Wheel Angle) -> [SteeringWheelAngle]
  [ResTorRight] -> Gain1/1
  [ResTorLeft] -> Gain2/1
  Gain1/1 -> Simulink-PS Converter1/1
  Gain2/1 -> Simulink-PS Converter2/1
  MATLAB Function/1(result) -> [WheelAngle_Left], Steering angle left/1
  MATLAB Function1/1(result) -> [WheelAngle_Right], Steering angle right/1
  Torque input/1 -> Gain/1
  "Sensing "/1(Steering angle left (rad)) -> MATLAB Function/1(input)
  PS-Simulink Converter1/1 -> "torque at "/1  "tc"
  PS-Simulink Converter/1 -> "torque at "/2  "tt"
  Gain/1 -> Simulink-PS Converter/1
  connections:
  Revolute/RConn2 -- "Sensing "/LConn2
  Simulink-PS Converter/RConn1 -- External Force and Torque/LConn1
  Chassis + Rack/LConn2 -- World/LConn1 -- Transform1/LConn1
  Rack and Pinion Constraint/RConn1 -- Chassis + Rack/LConn1
  Revolute1/RConn2 -- "Sensing "/LConn1
  Rack and Pinion Constraint/LConn1 -- pinion_1_RIGID/LConn2
  Transform1/RConn1 -- Stability Bar/LConn2
  Chassis + Rack/LConn3 -- pinion_1_RIGID/RConn1 -- External Force and Torque/RConn1
  Chassis + Rack/RConn1 -- Wheel Right/LConn1
  Revolute1/RConn1 -- Wheel Left/LConn1
  Chassis + Rack/RConn2 -- Wheel Left/LConn2
  Revolute1/LConn1 -- Stability Bar/RConn1
  Revolute/RConn1 -- Stability Bar/LConn1
  Revolute/LConn1 -- Wheel Right/RConn1
  Rod_2_RIGID/RConn1 -- pinion_1_RIGID/LConn3
  Steering_wheel/LConn1 -- Rod_2_RIGID/LConn1
  Revolute/RConn3 -- PS-Simulink Converter1/LConn1
  Revolute/RConn4 -- PS-Simulink Converter/LConn1

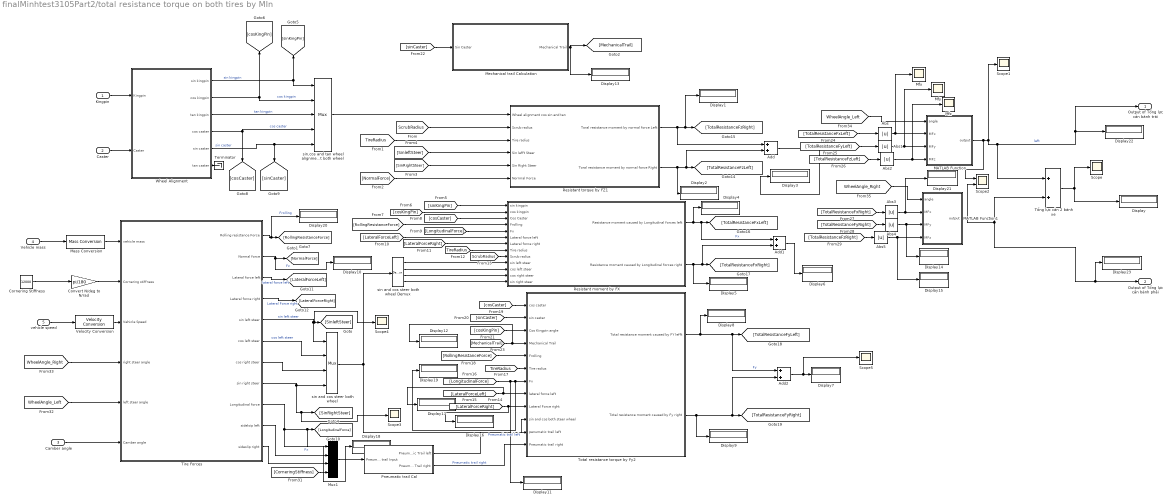
== system finalMinhtest3105Part2/total resistance torque on both tires by MIn ==
  Kingpin : Inport
  Caster : Inport  Port=2
  Camber angle : Inport  Port=3
  Vehicle mass : Inport  Port=4
  "vehicle speed " : Inport  Port=5
  Abs{,1..5} (6 alike) : Abs  SaturateOnIntegerOverflow=off
  Add : Sum
  Add1 : Sum
  Add2 : Sum
  Convert N/deg to N/rad : Gain  Gain=pi/180
  Cornering Stiffness : Constant  Value=12000
  Display{,1..23} (24 alike) : Display
  MATLAB Function : MATLAB Function  TreatAsAtomicUnit=on
  MATLAB Function1 : MATLAB Function  TreatAsAtomicUnit=on
  Mass Conversion : aerolibconvert2/Mass Conversion  IU=kg  OU=kg
  "Mechanical trail Calculation " : Subsystem
  Mfx : Scope
  Mfy : Scope
  Mfz : Scope
  Mux1 : Mux
  Pneumatic trail Cal : Subsystem
  Resistant moment by FX : Subsystem
  Resistant torque by FZ1 : Subsystem
  Scope{,1,3..5} (5 alike) : Scope
  Scope2 : Scope  NumInputPorts=2
  Terminator : Terminator
  Tire Forces : Subsystem
  Total resistance torque by Fy2 : Subsystem
  Tổng lực cản 2 bánh xe : Sum
  Velocity Conversion : aerolibconvert2/Velocity Conversion  IU=km/h  OU=m/s
  Wheel Alignment : Subsystem
  sin and cos steer both wheel : Mux
  sin and cos steer both wheel Demux : Demux
  sin,cos and tan wheel alignment both wheel : Mux  Inputs=5
  Output of Tổng lực cản bánh trái : Outport
  Output of Tổng lực cản bánh phải : Outport  Port=2
  wires:
  Kingpin/1 -> Wheel Alignment/1(Kingpin)
  Wheel Alignment/6(tan caster) -> Terminator/1
  Vehicle mass/1 -> Mass Conversion/1
  Mass Conversion/1 -> Tire Forces/1(vehicle mass)
  Cornering Stiffness/1 -> Convert N/deg to N/rad/1
  Caster/1 -> Wheel Alignment/2(Caster)
  "vehicle speed "/1 -> Velocity Conversion/1
  [WheelAngle_Right] -> Tire Forces/4("right steer angle ")
  [WheelAngle_Left] -> Tire Forces/5("left steer angle ")
  Velocity Conversion/1 -> Tire Forces/3(Vehicle Speed)
  Tire Forces/11(sideslip right) -> Mux1/3
  Tire Forces/10(sidelsip left) -> Mux1/2
  Tire Forces/9(Longitudinal force) -> Mux1/1, Display18/1, [LongitudinalForce]  "Fx"
  Mux1/1 -> Pneumatic trail Cal/1(Pneumatic trail Input)
  Pneumatic trail Cal/2(Pneumatic Trail right) -> Total resistance torque by Fy2/12(Pneumatic trail right)  "Pneumatic trail right"
  Pneumatic trail Cal/1(Pneumatic Trail left) -> Total resistance torque by Fy2/11(penumatic trail left)  "Pneumatic trail left"
  Tire Forces/5(sin left steer) -> sin and cos steer both wheel/1, Scope4/1, [SinleftSteer]  "sin left steer"
  Tire Forces/6(cos left steer) -> sin and cos steer both wheel/2  "cos left steer"
  Tire Forces/7(cos right steer) -> sin and cos steer both wheel/3
  Tire Forces/8(sin right steer) -> Scope3/1, [SinRightSteer], sin and cos steer both wheel/4
  sin and cos steer both wheel/1 -> Total resistance torque by Fy2/10(sin and cos both steer wheel), sin and cos steer both wheel Demux/1
  Wheel Alignment/1(sin kingpin) -> sin,cos and tan wheel alignment both wheel/1, [sinKingPin]  "sin kingpin"
  Wheel Alignment/2(cos kingpin) -> [cosKingPin], sin,cos and tan wheel alignment both wheel/2  "cos kingpin"
  Wheel Alignment/3(tan kingpin) -> sin,cos and tan wheel alignment both wheel/3  "tan kingpin"
  Wheel Alignment/4(cos caster) -> sin,cos and tan wheel alignment both wheel/4, [cosCaster]  "cos caster"
  Wheel Alignment/5(sin caster) -> [sinCaster], sin,cos and tan wheel alignment both wheel/5  "sin caster"
  sin,cos and tan wheel alignment both wheel/1 -> Resistant torque by FZ1/1("Wheel alignment cos sin and tan ")
  Tire Forces/2(Normal force) -> Display10/1, [NormalForce]  "Fz"
  [ScrubRadius] -> Resistant torque by FZ1/2(Scrub radius)
  [TireRadius] -> Resistant torque by FZ1/3(Tire radius)
  [sinKingPin] -> Resistant moment by FX/1(sin kingpin)
  [cosKingPin] -> Resistant moment by FX/2(cos kingpin)
  Tire Forces/1(Rolling resistance Force) -> Display20/1, [RollingResistanceForce]  "Frolling"
  [RollingResistanceForce] -> Resistant moment by FX/4(Frolling)
  [cosCaster] -> Resistant moment by FX/3(Cos Caster)
  [LongitudinalForce] -> Resistant moment by FX/5(Fx)
  Tire Forces/3(Lateral force left) -> [LateralForceLeft]  "lateral force left"
  Tire Forces/4(Lateral force right) -> [LateralForceRight]  "Lateral Force right"
  [LateralForceLeft] -> Resistant moment by FX/6(Lateral force left)
  [LateralForceRight] -> Resistant moment by FX/7(Lateral force right)
  [TireRadius] -> Resistant moment by FX/8(Tire radius)
  [ScrubRadius] -> Resistant moment by FX/9(Scrub radius)
  [LateralForceRight] -> Display16/1, Total resistance torque by Fy2/9(Lateral Force right)
  [TireRadius] -> Total resistance torque by Fy2/6(Tire radius)
  [RollingResistanceForce] -> Total resistance torque by Fy2/5(Frolling)
  [cosCaster] -> Total resistance torque by Fy2/1(cos caster)
  sin and cos steer both wheel Demux/1 -> Resistant moment by FX/10(sin left steer)
  sin and cos steer both wheel Demux/2 -> Resistant moment by FX/11(cos left steer)
  sin and cos steer both wheel Demux/3 -> Resistant moment by FX/12(cos right steer)
  sin and cos steer both wheel Demux/4 -> Resistant moment by FX/13(sin right steer)
  Resistant moment by FX/1(Resistance moment caused by Longitudinal forces left) -> Display4/1, Add1/1, [TotalResistanceFxLeft]  "Fx"
  Resistant moment by FX/2(Resistance moment caused by Longitudinal forces right) -> Display5/1, Add1/2, [TotalResistanceFxRight]
  Total resistance torque by Fy2/2(Total resistance moment caused by Fy right) -> Display9/1, Add2/2, [TotalResistanceFyRight]
  Total resistance torque by Fy2/1("Total resistance moment caused by FY lefft ") -> Display8/1, Add2/1, [TotalResistanceFyLeft]  "Fy"
  [TotalResistanceFxLeft] -> Abs/1
  [TotalResistanceFyLeft] -> Abs1/1
  [TotalResistanceFzLeft] -> Abs2/1
  [TotalResistanceFxRight] -> Abs3/1
  [TotalResistanceFyRight] -> Abs4/1
  [TotalResistanceFzRight] -> Abs5/1
  Tổng lực cản 2 bánh xe/1 -> Scope/1, Display/1
  Convert N/deg to N/rad/1 -> Tire Forces/2(Cornering stiffness)
  [CorneringStiffness] -> Mux1/4
  [sinCaster] -> Total resistance torque by Fy2/2(sin caster)
  [cosKingPin] -> Total resistance torque by Fy2/3(Cos Kingpin angle)
  [MechanicalTrail] -> Display12/1, Total resistance torque by Fy2/4(Mechanical Trail)
  [LongitudinalForce] -> Display19/1, Total resistance torque by Fy2/7(Fx), Display11/1
  [LateralForceLeft] -> Display17/1, Total resistance torque by Fy2/8(lateral force left)
  [SinleftSteer] -> Resistant torque by FZ1/4(Sin lefft Steer)
  [SinRightSteer] -> Resistant torque by FZ1/5(Sin Right Steer)
  [NormalForce] -> Resistant torque by FZ1/6(Norrmal Force)
  Resistant torque by FZ1/1(Toral resistance moment by normal force Left) -> Add/1, Display1/1, [TotalResistanceFzRight]
  Resistant torque by FZ1/2(Toral resistance moment by normal force Right) -> Display2/1, Add/2, [TotalResistanceFzLeft]
  Add/1 -> Display3/1
  Add1/1 -> Display6/1
  Add2/1 -> Scope5/1, Display7/1
  "Mechanical trail Calculation "/1(Mechanical Trail) -> [MechanicalTrail], Display13/1
  [sinCaster] -> "Mechanical trail Calculation "/1(Sin Caster)
  Camber angle/1 -> Tire Forces/6(Camber angle)
  MATLAB Function/1(output) -> Scope2/1, Output of Tổng lực cản bánh trái/1, Display22/1, Tổng lực cản 2 bánh xe/1, Scope1/1  "left"
  [WheelAngle_Left] -> MATLAB Function/1(angle)
  MATLAB Function1/1(output) -> Scope2/2, Display23/1, Output of Tổng lực cản bánh phải/1, Tổng lực cản 2 bánh xe/2
  [WheelAngle_Right] -> MATLAB Function1/1(angle)
  Abs/1 -> MATLAB Function/2(MFx), Mfx/1
  Abs1/1 -> MATLAB Function/3(MFy), Mfy/1
  Abs2/1 -> Mfz/1, MATLAB Function/4(MFz)
  Abs3/1 -> Display21/1, MATLAB Function1/2(MFx)
  Abs4/1 -> Display14/1, MATLAB Function1/3(MFy)
  Abs5/1 -> Display15/1, MATLAB Function1/4(MFz)

== system finalMinhtest3105Part2/Steering Dynamics/Chassis + Rack ==
  Add : Sum
  Constant : Constant  Value=2.73
  Gain : Gain  Gain=-5.4
  Rack Case + Chassis : Subsystem
  Rack_1_RIGID : Subsystem
  Radians to Degrees : simulink_extras/Transformations/Radians to Degrees
  Target : PMIOPort  Side=Left
  Conn3 : PMIOPort  Port=2  Side=Left
  Conn1 : PMIOPort  Port=3  Side=Left
  F2 : PMIOPort  Port=4  Side=Right
  F3 : PMIOPort  Port=5  Side=Right
  Steering Wheel Angle : Outport
  Steering Wheel Velocity : Outport  Port=2
  wires:
  Rack Case + Chassis/1(Steering Wheel Angle) -> Add/1
  Constant/1 -> Add/2
  Add/1 -> Radians to Degrees/1
  Radians to Degrees/1 -> Gain/1
  Gain/1 -> Steering Wheel Angle/1
  Rack Case + Chassis/2(Steering Wheel Velocity) -> Steering Wheel Velocity/1
  connections:
  Rack_1_RIGID/RConn1 -- Rack Case + Chassis/LConn2
  Rack_1_RIGID/RConn2 -- Rack Case + Chassis/LConn3
  Rack_1_RIGID/RConn4 -- Rack Case + Chassis/LConn5
  Conn3/RConn1 -- Rack Case + Chassis/LConn1
  Target/RConn1 -- Rack_1_RIGID/LConn1
  Rack Case + Chassis/LConn4 -- Rack_1_RIGID/RConn3
  Rack Case + Chassis/LConn7 -- F2/RConn1
  Rack Case + Chassis/LConn6 -- Rack_1_RIGID/RConn5
  Rack Case + Chassis/RConn2 -- F3/RConn1
  Rack Case + Chassis/RConn1 -- Conn1/RConn1

== system finalMinhtest3105Part2/Steering Dynamics/Rod_2_RIGID ==
  ReferenceFrame : sm_lib/Frames and Transforms/Reference Frame
  Solid : sm_lib/Body Elements/File Solid  ExtGeomFileName=Rod_Default_sldprt.STEP  UnitType=FromFile  ExtGeomFileUnits=m  StepReaderType=HEX  ExportConvexHullGeometry=off  InertiaType=Custom  Mass=smiData.Solid(4).mass  MassUnits=kg  CenterOfMass=smiData.Solid(4).CoM  CenterOfMassUnits=mm  MomentsOfInertia=smiData.Solid(4).MoI  MomentsOfInertiaUnits=kg*mm^2  ProductsOfInertia=smiData.Solid(4).PoI  ProductsOfInertiaUnits=kg*mm^2  BasedOnType=DensityFromFile  Density=1000  DensityUnits=kg/m^3  DoExposeReferenceFrame=on  SerializedFrames=<Frames/>  GraphicType=FromGeometry  MarkerShape=Sphere  MarkerSize=10  GraphicVisPropType=SimpleVisualProperties  GraphicDiffuseColor=smiData.Solid(4).color  GraphicSpecularColor=[0.5 0.5 0.5 1.0]  GraphicAmbientColor=[0.15 0.15 0.15 1.0]  GraphicEmissiveColor=[0.0 0.0 0.0 1.0]  GraphicShininess=75  GraphicOpacity=smiData.Solid(4).opacity
  Transform : sm_lib/Frames and Transforms/Rigid Transform  TranslationMethod=Cartesian  TranslationStandardOffset=0  TranslationLengthUnit=mm  TranslationStandardAxis=+Z  TranslationCartesianOffset=smiData.RigidTransform(39).translation  TranslationROffset=0  TranslationROffsetUnits=m  TranslationZOffset=0  TranslationZOffsetUnits=m  TranslationThetaOffset=0  TranslationThetaOffsetUnits=deg  RotationMethod=ArbitraryAxis  RotationAngleUnits=rad  RotationStandardAxis=+Z  RotationAngle=smiData.RigidTransform(39).angle  RotationArbitraryAxis=smiData.RigidTransform(39).axis  FollAlignAxisA=+X  BaseAlignAxisA=+Y  FollAlignAxisB=+Y  BaseAlignAxisB=+Z  RotationSequenceAxes=FollowerAxes  RotationSequence=XYX  RotationSequenceAngles=[0 0 0]  RotationSequenceAnglesUnits=deg  RotationMatrix=[1 0 0; 0 1 0; 0 0 1]  Quaternion=[1 0 0 0]
  Transform1 : sm_lib/Frames and Transforms/Rigid Transform  TranslationMethod=Cartesian  TranslationStandardOffset=0  TranslationLengthUnit=mm  TranslationStandardAxis=+Z  TranslationCartesianOffset=smiData.RigidTransform(42).translation  TranslationROffset=0  TranslationROffsetUnits=m  TranslationZOffset=0  TranslationZOffsetUnits=m  TranslationThetaOffset=0  TranslationThetaOffsetUnits=deg  RotationMethod=ArbitraryAxis  RotationAngleUnits=rad  RotationStandardAxis=+Z  RotationAngle=smiData.RigidTransform(42).angle  RotationArbitraryAxis=smiData.RigidTransform(42).axis  FollAlignAxisA=+X  BaseAlignAxisA=+Y  FollAlignAxisB=+Y  BaseAlignAxisB=+Z  RotationSequenceAxes=FollowerAxes  RotationSequence=XYX  RotationSequenceAngles=[0 0 0]  RotationSequenceAnglesUnits=deg  RotationMatrix=[1 0 0; 0 1 0; 0 0 1]  Quaternion=[1 0 0 0]
  F : PMIOPort  Side=Left
  F1 : PMIOPort  Port=2  Side=Right
  connections:
  Solid/RConn1 -- ReferenceFrame/RConn1 -- Transform/LConn1 -- Transform1/LConn1
  Transform/RConn1 -- F/RConn1
  Transform1/RConn1 -- F1/RConn1
